simulink library "limblab"  (R2015a)
settings: Solver=ode45  SolverMode=SingleTasking  StartTime=0.0  StopTime=10.0  RelTol=1e-3
undefined symbols (not defined in the file or in its folder): dfilt
libraries: simulink x24, limblab x9, xpcnilib x5, slrtlib x4, dspobslib x4, xpcrtudplib x3, xpcobsoletelib x3, dspsigops x2, xpcmeasurementcomputinglib x2, simulink_extras x1
(part 2 of 2)

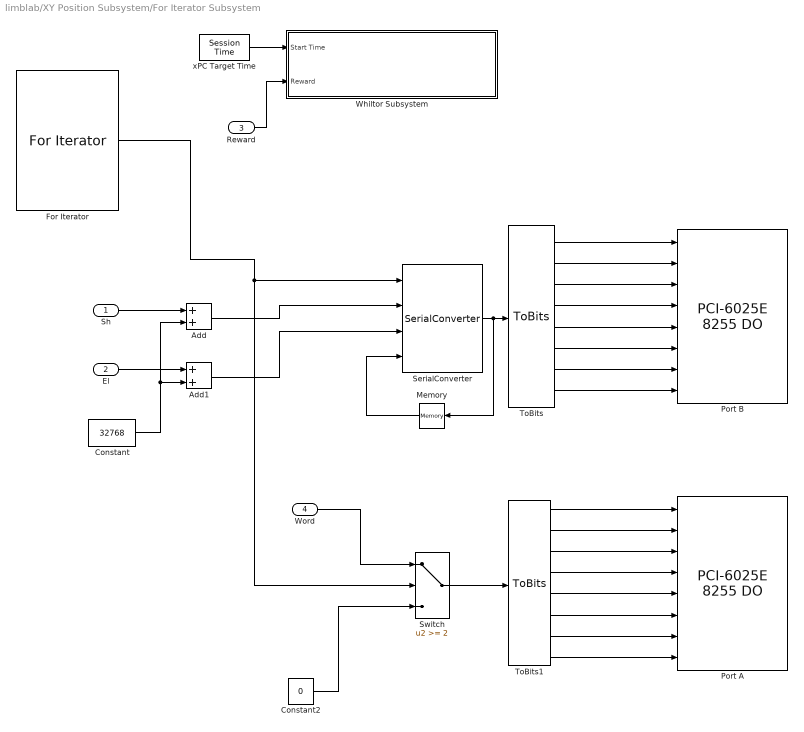
== system limblab/XY Position Subsystem/For Iterator Subsystem ==
  Sh : Inport
  "El " : Inport  Port=2
  Reward : Inport  Port=3
  Word : Inport  Port=4
  Add : Sum
  Add1 : Sum
  Constant : Constant  Value=32768
  Constant2 : Constant  Value=0
  For Iterator : ForIterator  IndexMode=Zero-based  IterationVariableDataType=double
  Memory : Memory  InheritSampleTime=on
  Port A : xpcnilib/Digital Output/E Series/PCI-6025E 8255 DO  channel=1:8  port=A  reset=[1]  initValue=[0]  chip=1  sampletime=-1  slot=-1
  Port B : xpcnilib/Digital Output/E Series/PCI-6025E 8255 DO  channel=1:8  port=B  reset=[1]  initValue=[0]  chip=1  sampletime=-1  slot=-1
  SerialConverter : limblab/SerialConverter
  Switch : Switch  Threshold=2
  ToBits : limblab/ToBits
  ToBits1 : limblab/ToBits
  Whiltor Subsystem : Subsystem  TreatAsAtomicUnit=on
  "xPC Target Time " : slrtlib/Target Management/Target Information/Session Time   ts=-1
  wires:
  "xPC Target Time "/1 -> Whiltor Subsystem/1(Start Time)
  SerialConverter/1 -> Memory/1, ToBits/1
  Sh/1 -> Add/1
  Add/1 -> SerialConverter/2
  Add1/1 -> SerialConverter/3
  "El "/1 -> Add1/1
  Constant/1 -> Add/2, Add1/2
  ToBits/1 -> Port B/1
  ToBits/2 -> Port B/2
  ToBits/3 -> Port B/3
  ToBits/4 -> Port B/4
  ToBits/5 -> Port B/5
  ToBits/6 -> Port B/6
  ToBits/7 -> Port B/7
  ToBits/8 -> Port B/8
  Reward/1 -> Whiltor Subsystem/2(Reward)
  ToBits1/1 -> Port A/1
  ToBits1/2 -> Port A/2
  ToBits1/3 -> Port A/3
  ToBits1/4 -> Port A/4
  ToBits1/5 -> Port A/5
  ToBits1/6 -> Port A/6
  ToBits1/7 -> Port A/7
  ToBits1/8 -> Port A/8
  Constant2/1 -> Switch/3
  Word/1 -> Switch/1
  Switch/1 -> ToBits1/1
  For Iterator/1 -> SerialConverter/1, Switch/2
  Memory/1 -> SerialConverter/4

== system limblab/XY Position Subsystem/Handle Rotation ==
  Xin : Inport
  Yin : Inport  Port=2
  ElbowAngle : Inport  Port=3
  Mux : Mux  Inputs=2
  Product : Product  RndMeth=Zero
  Product1 : Product  RndMeth=Zero
  Sum : Sum  Inputs=|++
  Trigonometric Function : Trigonometry
  Trigonometric Function1 : Trigonometry  Operator=atan2
  Trigonometric Function2 : Trigonometry  Operator=cos
  sqrt(u[1]*u[1] + u[2]*u[2]) : Fcn  Expr=sqrt(u[1]*u[1] + u[2]*u[2])
  Xout : Outport
  Yout : Outport  Port=2
  wires:
  ElbowAngle/1 -> Sum/2
  Trigonometric Function1/1 -> Sum/1
  Xin/1 -> Mux/2, Trigonometric Function1/2
  Mux/1 -> sqrt(u[1]*u[1] + u[2]*u[2])/1
  Trigonometric Function/1 -> Product/2
  Product/1 -> Yout/1
  sqrt(u[1]*u[1] + u[2]*u[2])/1 -> Product/1, Product1/2
  Sum/1 -> Trigonometric Function/1, Trigonometric Function2/1
  Product1/1 -> Xout/1
  Trigonometric Function2/1 -> Product1/1
  Yin/1 -> Mux/1, Trigonometric Function1/1

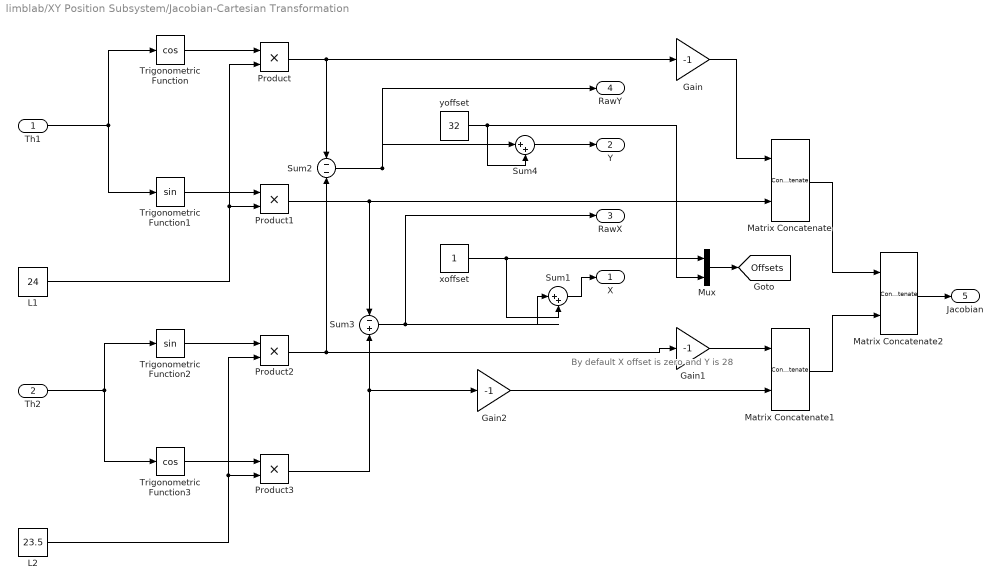
== system limblab/XY Position Subsystem/Jacobian-Cartesian Transformation ==
  note: By default X offset is zero and Y is 28
  Th1 : Inport
  Th2 : Inport  Port=2
  Gain : Gain  Gain=-1
  Gain1 : Gain  Gain=-1
  Gain2 : Gain  Gain=-1
  L1 : Constant  Value=24
  L2 : Constant  Value=23.5
  Matrix Concatenate : Concatenate  ConcatenateDimension=2
  Matrix Concatenate1 : Concatenate  ConcatenateDimension=2
  Matrix Concatenate2 : Concatenate  Mode=Multidimensional array  ConcatenateDimension=2
  Mux : Mux  Inputs=2
  Product{,1..3} (4 alike) : Product  RndMeth=Zero
  Sum1 : Sum  Inputs=|++  SaturateOnIntegerOverflow=on  InputSameDT=on  OutDataTypeStr=Inherit: Same as first input
  Sum2 : Sum  Inputs=--  SaturateOnIntegerOverflow=on  InputSameDT=on  OutDataTypeStr=Inherit: Same as first input
  Sum3 : Sum  Inputs=-+  SaturateOnIntegerOverflow=on  InputSameDT=on  OutDataTypeStr=Inherit: Same as first input
  Sum4 : Sum  Inputs=|++  SaturateOnIntegerOverflow=on  InputSameDT=on  OutDataTypeStr=Inherit: Same as first input
  Trigonometric Function : Trigonometry  Operator=cos
  Trigonometric Function1 : Trigonometry
  Trigonometric Function2 : Trigonometry
  Trigonometric Function3 : Trigonometry  Operator=cos
  xoffset : Constant
  yoffset : Constant  Value=32
  X : Outport
  Y : Outport  Port=2
  RawX : Outport  Port=3
  RawY : Outport  Port=4
  Jacobian : Outport  Port=5
  tag scope: Offsets=global
  wires:
  Th1/1 -> Trigonometric Function/1, Trigonometric Function1/1
  Product/1 -> Sum2/1, Gain/1
  Product2/1 -> Sum2/2, Gain1/1
  Product1/1 -> Sum3/1, Matrix Concatenate/2
  Sum2/1 -> RawY/1, Sum4/1
  Sum4/1 -> Y/1
  Sum1/1 -> X/1
  xoffset/1 -> Sum1/2, Mux/1
  yoffset/1 -> Sum4/2, Mux/2
  Product3/1 -> Gain2/1, Sum3/2
  Th2/1 -> Trigonometric Function2/1, Trigonometric Function3/1
  Matrix Concatenate/1 -> Matrix Concatenate2/1
  Matrix Concatenate1/1 -> Matrix Concatenate2/2
  Matrix Concatenate2/1 -> Jacobian/1
  Gain/1 -> Matrix Concatenate/1
  Gain1/1 -> Matrix Concatenate1/1
  Gain2/1 -> Matrix Concatenate1/2
  Trigonometric Function/1 -> Product/1
  Trigonometric Function3/1 -> Product3/1
  Trigonometric Function2/1 -> Product2/1
  L2/1 -> Product3/2, Product2/2
  Trigonometric Function1/1 -> Product1/1
  L1/1 -> Product/2, Product1/2
  Mux/1 -> [Offsets]
  Sum3/1 -> RawX/1, Sum1/1

== system limblab/XY Position Subsystem/OffsetCalculation ==
  RawForce : Inport
  Abs : Abs
  Add : Sum  Inputs=+-
  Compare To Constant1 : simulink/Logic and Bit Operations/Compare To Constant  relop=>=  const=1000  OutDataTypeStr=boolean
  Discrete-Time Integrator : DiscreteIntegrator  IntegratorMethod=Accumulation: Forward Euler  gainval=1  ExternalReset=falling  SampleTime=-1  OutDataTypeStr=int32  LimitOutput=on  UpperSaturationLimit=1000  LowerSaturationLimit=-1
  F Offset : Constant  Value=[-.73 .08 .21 -.23 .25 .44]  VectorParams1D=off  SampleTime=-1
  Gain : Gain  Gain=49
  Gain1 : Gain  Gain=1/50
  Memory : Memory
  NoiseLevel : simulink/Logic and Bit Operations/Compare To Constant  relop=<=  const=.03  OutDataTypeStr=uint8
  Sum : Sum  Inputs=|++
  Sum of Elements : Sum  Inputs=+
  Switch : Switch
  Unit Delay1 : UnitDelay  SampleTime=.001
  Offsets : Outport
  wires:
  RawForce/1 -> Sum/1, Add/1
  Add/1 -> Abs/1
  Abs/1 -> Sum of Elements/1
  Sum of Elements/1 -> NoiseLevel/1
  NoiseLevel/1 -> Discrete-Time Integrator/2, Discrete-Time Integrator/1
  Unit Delay1/1 -> Gain/1
  Sum/1 -> Gain1/1
  Gain1/1 -> Switch/1, Unit Delay1/1, Add/2
  Discrete-Time Integrator/1 -> Compare To Constant1/1
  Compare To Constant1/1 -> Switch/2
  Switch/1 -> Memory/1, Offsets/1
  Memory/1 -> Switch/3
  Gain/1 -> Sum/2

== system limblab/Motor Control/Schmidt/Enabled Subsystem ==
  In1 : Inport
  Enable : EnablePort
  Out1 : Outport
  wires:
  In1/1 -> Out1/1

== system limblab/Recentering Subsystem/Schmidt1/Enabled Subsystem ==
  In1 : Inport
  Enable : EnablePort
  Out1 : Outport
  wires:
  In1/1 -> Out1/1

== system limblab/Recentering Subsystem/Schmidt2/Enabled Subsystem ==
  In1 : Inport
  Enable : EnablePort
  Out1 : Outport
  wires:
  In1/1 -> Out1/1

== system limblab/Recentering Subsystem/Schmidt3/Enabled Subsystem ==
  In1 : Inport
  Enable : EnablePort
  Out1 : Outport
  wires:
  In1/1 -> Out1/1

== system limblab/XY Position Subsystem/For Iterator Subsystem/Whiltor Subsystem ==
  Start Time : Inport
  Reward : Inport  Port=2
  Compare To Constant : simulink/Logic and Bit Operations/Compare To Constant  relop=<=  const=125  OutDataTypeStr=boolean
  Compare To Constant1 : simulink/Logic and Bit Operations/Compare To Constant  relop=>  const=100  OutDataTypeStr=boolean  ZeroCross=off
  Constant : Constant
  Constant1 : Constant  Value=0
  "PCI-6025E " : xpcnilib/Digital Output/E Series/PCI-6025E DO  channel=[1 2]  reset=[1]  initValue=[0]  sampletime=-1  slot=-1
  ScaleTouSec : Gain  Gain=.838
  Subtract : Sum  Inputs=+-
  Switch : Switch  Criteria=u2 ~= 0
  While Iterator : WhileIterator  MaxIters=-1  WhileBlockType=do-while
  "xPC Target Time " : slrtlib/Target Management/Target Information/Session Time   ts=-1
  wires:
  "xPC Target Time "/1 -> Subtract/1
  Start Time/1 -> Subtract/2
  Subtract/1 -> ScaleTouSec/1
  Compare To Constant/1 -> While Iterator/1
  ScaleTouSec/1 -> Compare To Constant/1, Compare To Constant1/1
  Compare To Constant1/1 -> Switch/2
  Constant/1 -> Switch/1
  Constant1/1 -> Switch/3
  Switch/1 -> "PCI-6025E "/1
  Reward/1 -> "PCI-6025E "/2
